simulink model "mass_spring"  (R2021a)
settings: Solver=VariableStepAuto  StartTime=0.0  StopTime=10.0  RelTol=1e-3
settings Model: Creator=Beshary  LastModifiedBy=Beshary

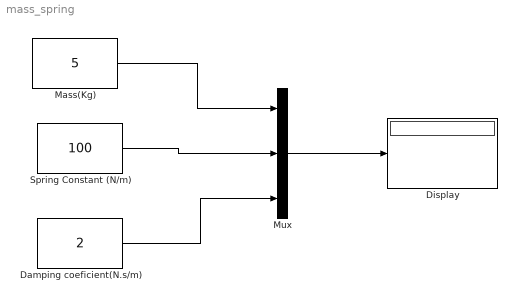
== system mass_spring ==
  Damping coeficient(N.s/m) : Constant  Value=2
  Display : Display
  Mass(Kg) : Constant  Value=5
  Mux : Mux  Inputs=3
  Spring Constant (N/m) : Constant  Value=100
  wires:
  Mass(Kg)/1 -> Mux/1
  Damping coeficient(N.s/m)/1 -> Mux/3
  Spring Constant (N/m)/1 -> Mux/2
  Mux/1 -> Display/1
